simulink model "practice9__1"  (Simulink 7.9)
settings: Solver=ode45  StartTime=0.0  StopTime=10.0  RelTol=1e-3
settings Model: Creator=sony  LastModifiedBy=sony

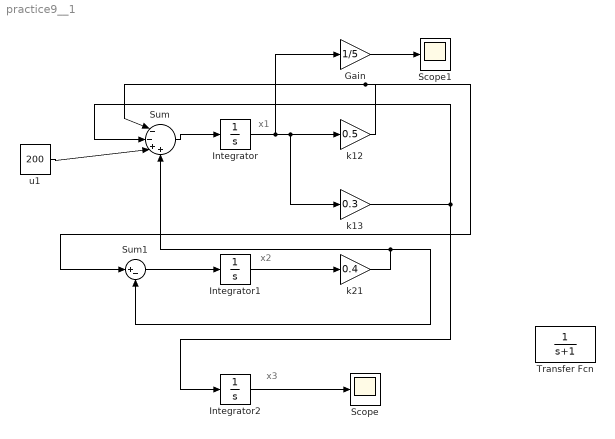
== system practice9__1 ==
  note: x1
  note: x2
  note: x3
  Gain : Gain  Gain=1/5
  Integrator : Integrator
  Integrator1 : Integrator
  Integrator2 : Integrator
  Scope : Scope
  Scope1 : Scope
  Sum : Sum  Inputs=|--++
  Sum1 : Sum  Inputs=|+-
  Transfer Fcn : TransferFcn  Denominator=[1 1]
  k12 : Gain  Gain=0.5
  k13 : Gain  Gain=0.3
  k21 : Gain  Gain=0.4
  u1 : Constant  Value=200
  wires:
  Integrator/1 -> k12/1, k13/1, Gain/1
  Integrator1/1 -> k21/1
  k12/1 -> Sum/1, Sum1/1
  k13/1 -> Sum/2, Integrator2/1
  u1/1 -> Sum/3
  Sum/1 -> Integrator/1
  k21/1 -> Sum/4, Sum1/2
  Sum1/1 -> Integrator1/1
  Integrator2/1 -> Scope/1
  Gain/1 -> Scope1/1
